simulink model "TanquesAcoplados"  (R2016a)
settings: Solver=VariableStepAuto  StartTime=0.0  StopTime=500  RelTol=1e-3
values from neighbouring files (symbols this model uses):
  A = [double(subs(df1_dh1)) double(subs(df1_dh2)) ... (first row only)    [ModeloLinear.m]
  B = [double(subs(df1_dq1)) double(subs(df1_dq2)) ... (first row only)    [ModeloLinear.m]
  C = [1 0;0 1]    [ModeloLinear.m]
  D = [0 0; 0 0]    [ModeloLinear.m]
  H1 = 25    [ModeloLinear.m]
  H2 = 21    [ModeloLinear.m]
  K1 = 25    [ModeloLinear.m]
  K2 = K1    (= 25)    [ModeloLinear.m]
  Q1 = 100    [ModeloLinear.m]
  Q2 = 90    [ModeloLinear.m]
settings Model: Creator=JesseAlves  LastModifiedBy=JesseAlves

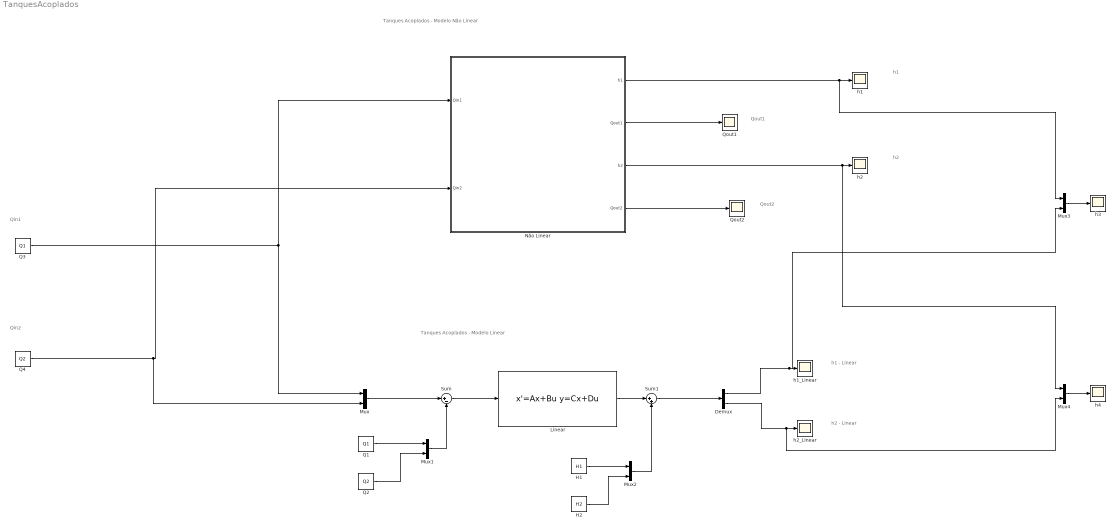
== system TanquesAcoplados ==
  note: Tanques Acoplados - Modelo Não Linear
  note: Qin1
  note: Qin2
  note: h1
  note: Qout2
  note: Qout1
  note: h2
  note: Tanques Acoplados - Modelo Linear
  note: h1 - Linear
  note: h2 - Linear
  Demux : Demux  Outputs=2
  H1 : Constant  Value=H1
  H2 : Constant  Value=H2
  Linear : StateSpace  A=A  B=B  C=C  D=D  X0=0
  Mux{,1..4} (5 alike) : Mux  Inputs=2
  Não Linear : Subsystem
  Q1 : Constant  Value=Q1
  Q2 : Constant  Value=Q2
  Q3 : Constant  Value=Q1
  Q4 : Constant  Value=Q2
  Qout1 : Scope
  Qout2 : Scope
  Sum : Sum  Inputs=|+-
  Sum1 : Sum  Inputs=|++
  h{1..4} (4 alike) : Scope
  "h1_Linear " : Scope
  h2_Linear : Scope
  wires:
  Não Linear/1(h1) -> Mux3/1, h1/1
  Não Linear/2(Qout1) -> Qout1/1
  Não Linear/4(Qout2) -> Qout2/1
  Sum/1 -> Linear/1
  Linear/1 -> Sum1/1
  Q1/1 -> Mux1/1
  Q2/1 -> Mux1/2
  Mux1/1 -> Sum/2
  Mux/1 -> Sum/1
  H1/1 -> Mux2/1
  Mux2/1 -> Sum1/2
  H2/1 -> Mux2/2
  Sum1/1 -> Demux/1
  Demux/1 -> Mux3/2, "h1_Linear "/1
  Mux3/1 -> h3/1
  Não Linear/3(h2) -> Mux4/1, h2/1
  Demux/2 -> Mux4/2, h2_Linear/1
  Mux4/1 -> h4/1
  Q3/1 -> Não Linear/1(Qin1), Mux/1
  Q4/1 -> Mux/2, Não Linear/2(Qin2)

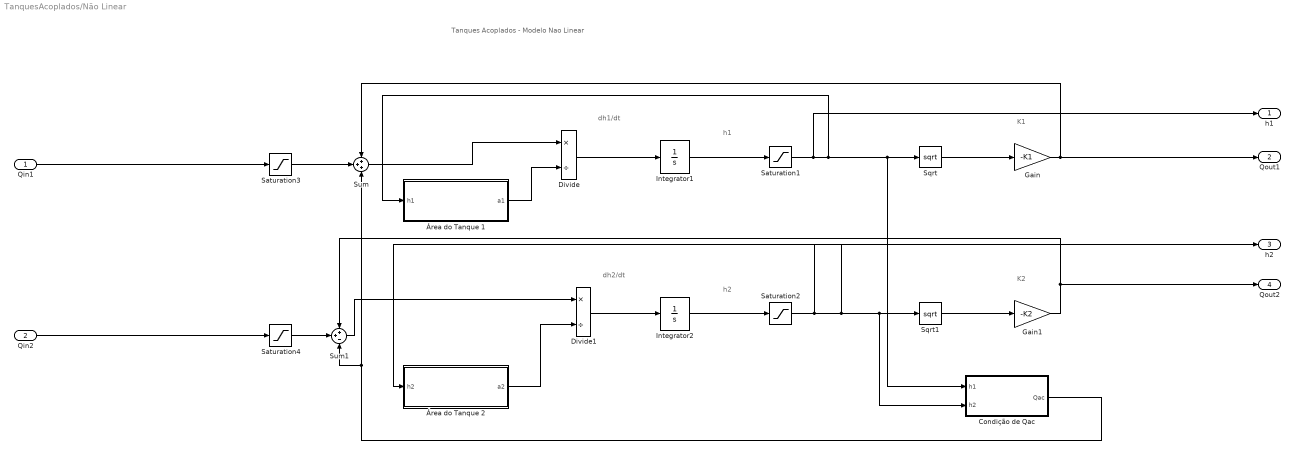
== system TanquesAcoplados/Não Linear ==
  note: h1
  note: h2
  note: dh1/dt
  note: dh2/dt
  note: K1
  note: K2
  note: Tanques Acoplados - Modelo Nao Linear
  Qin1 : Inport
  Qin2 : Inport  Port=2
  Condição de Qac : MATLAB Function  TreatAsAtomicUnit=on
  Divide : Product  Inputs=*/
  Divide1 : Product  Inputs=*/
  Gain : Gain  Gain=-K1
  Gain1 : Gain  Gain=-K2
  Integrator1 : Integrator
  Integrator2 : Integrator
  Saturation1 : Saturate  UpperLimit=49  LowerLimit=0
  Saturation2 : Saturate  UpperLimit=49  LowerLimit=0
  Saturation3 : Saturate  UpperLimit=160  LowerLimit=0
  Saturation4 : Saturate  UpperLimit=160  LowerLimit=0
  Sqrt : Sqrt  SaturateOnIntegerOverflow=on
  Sqrt1 : Sqrt  SaturateOnIntegerOverflow=on
  Sum : Sum  Inputs=+++
  Sum1 : Sum  Inputs=++-
  Área do Tanque 1 : MATLAB Function  TreatAsAtomicUnit=on
  Área do Tanque 2 : MATLAB Function  TreatAsAtomicUnit=on
  h1 : Outport
  Qout1 : Outport  Port=2
  h2 : Outport  Port=3
  Qout2 : Outport  Port=4
  wires:
  Sqrt/1 -> Gain/1
  Gain/1 -> Qout1/1, Sum/1
  Condição de Qac/1(Qac) -> Sum1/3, Sum/3
  Gain1/1 -> Qout2/1, Sum1/1
  Saturation1/1 -> h1/1, Área do Tanque 1/1(h1), Sqrt/1, Condição de Qac/1(h1)
  Integrator1/1 -> Saturation1/1
  Integrator2/1 -> Saturation2/1
  Qin1/1 -> Saturation3/1
  Saturation3/1 -> Sum/2
  Sum1/1 -> Divide1/1
  Saturation4/1 -> Sum1/2
  Qin2/1 -> Saturation4/1
  Saturation2/1 -> h2/1, Área do Tanque 2/1(h2), Sqrt1/1, Condição de Qac/2(h2)
  Sqrt1/1 -> Gain1/1
  Divide/1 -> Integrator1/1
  Área do Tanque 1/1(a1) -> Divide/2
  Sum/1 -> Divide/1
  Divide1/1 -> Integrator2/1
  Área do Tanque 2/1(a2) -> Divide1/2

== matlab function TanquesAcoplados/Não Linear/Área do Tanque 1 ==
  data: h1 input; a1 output
% ==> Funcao para calcular valor de K_fi
function a1 = Variacao_Nivel(h1)
    A1 = area1(h1);    
a1 = A1;

== matlab function TanquesAcoplados/Não Linear/Condição de Qac ==
  data: h1 input; Qac output; h2 input
% ==> Funcao para calcular valor de K_fi
function Qac = acoplamento(h1,h2)
    Kac = 20;
    qac = 0;
    if h1 >= h2
        qac = -Kac*sqrt(abs(h1 - h2));
    elseif h1 < h2
        qac = Kac*sqrt(abs(h1 - h2));
    end
Qac = qac;

== matlab function TanquesAcoplados/Não Linear/Área do Tanque 2 ==
  data: h2 input; a2 output
% ==> Funcao para calcular valor de K_fi
function a2 = Variacao_Nivel2(h2)
    A2 = area2(h2);
a2 = A2;
